simulink model "ee105lab5pt2"  (R2016b)
settings: Solver=VariableStepAuto  StartTime=0.0  StopTime=0.8  FixedStep=0.001  RelTol=1e-3
settings Model: Creator=jesselayman  LastModifiedBy=jesselayman

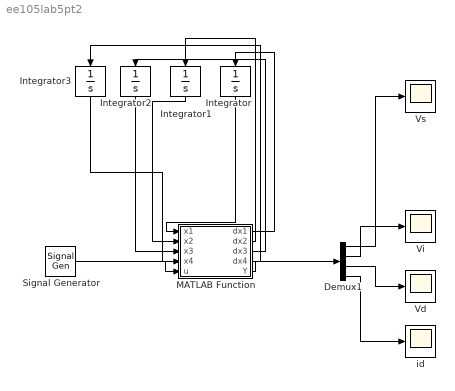
== system ee105lab5pt2 ==
  Demux1 : Demux
  Integrator{,1..3} (4 alike) : Integrator
  MATLAB Function : MATLAB Function  TreatAsAtomicUnit=on
  Signal Generator : SignalGenerator  Amplitude=120  Frequency=60
  Vd : Scope
  Vi : Scope
  "Vs " : Scope
  id : Scope
  wires:
  MATLAB Function/5(Y) -> Demux1/1
  MATLAB Function/1(dx1) -> Integrator/1
  Signal Generator/1 -> MATLAB Function/5(u)
  Integrator/1 -> MATLAB Function/1(x1)
  Demux1/1 -> "Vs "/1
  Demux1/2 -> Vi/1
  Demux1/3 -> Vd/1
  Demux1/4 -> id/1
  MATLAB Function/2(dx2) -> Integrator1/1
  Integrator1/1 -> MATLAB Function/2(x2)
  MATLAB Function/3(dx3) -> Integrator2/1
  Integrator2/1 -> MATLAB Function/3(x3)
  MATLAB Function/4(dx4) -> Integrator3/1
  Integrator3/1 -> MATLAB Function/4(x4)

== matlab function ee105lab5pt2/MATLAB Function ==
  data: x1 input; x2 input; x3 input; x4 input; u input; dx1 output; dx2 output; dx3 output; dx4 output; Y output

function [dx1,dx2,dx3,dx4,Y]= fxnblk(x1,x2,x3,x4,u) 
N = 10;
C = .0001;
R = 100;
L = 0.883; %Derived from graph part 1
Vd = u/N - x1;
id = diode(Vd);
%dx1..dx4 derived from state space model 
dx1 = 1/C*(id-x2);
dx2 = 1/L*(x1-x3); 
dx3 = 1/C*(x2-x4);
dx4 = 1/L*(x3-R*x4);
Y = [R*x4,x1,Vd,id];


end

%Diode function provided in the lab
function [id]=diode(vd) 
A = 0.0007;
if vd > 0.7
Rd = 0.01;
id = A + (vd - 0.7)/Rd; 


else
Rd = 1000;
id = A + (vd - 0.7)/Rd; 
end
end
